simulink model "Hexa_CAD_ANSFT_Sim_V3"  (R2023a)
settings: Solver=ode4  StartTime=0.0  StopTime=30  FixedStep=0.01  RelTol=1e-3
model workspace (MAT data in the model file):
  hover_2m = [0 0 2 0 0 0 0 0 2 0 0 0 ... (36 elements, 6x6)]
  square = [0 0 2.5 0 0 0 0 0 2.5 0 0 0 ... (36 elements, 6x6)]
  tf : Simulink.Parameter (value not decoded)
  tray0 = [0 0 0 0 0 0 0.2 0.15 2 0 0 0 ... (36 elements, 6x6)]
  tray1 = [0 0 0 0 0 0 0 0 2 0 0 0 ... (36 elements, 6x6)]
  tray2 = [0 0 0 0 0 0 2 0 5 0 0 0 ... (36 elements, 6x6)]
  tray3 = [0 0 0 0 0 0 2 0 5 0 0 0 ... (36 elements, 6x6)]
  tray4 = [0 0 0 0 0 0 2 0 5 0.15 0 0 ... (36 elements, 6x6)]
  tray5 = [0 0 0 0 0 0 0 0 5 0.15 0 0 ... (36 elements, 6x6)]
  tray_yaw = [0 0 0 0 0 0 0 0 5 0 0 0 ... (36 elements, 6x6)]
undefined symbols (not defined in the file or in its folder): F, Light, MIL, smiData, X, Y, Z
libraries: sm_lib x168, nesl_utility x33, dspsrcs4 x9, sharedtransform x3, simulink x3, robotcorelib x1, aerolibwind2 x1
(part 6 of 6)

== matlab function Hexa_CAD_ANSFT_Sim_V3/Trajectory/Helicoidal Trajectory ==
  data: time input; pose_d output; pose_d_dot output; pose_d_ddot output
function [pose_d, pose_d_dot, pose_d_ddot]= fcn(time)

% pos_z = time / 12;
f = 0.15;
arg = f * (time - 5);
r = 2;

% hover for 5 s | include inclination in roll
% 5 metros al menos

roll = 0;
% yaw = pi / 2;
yaw = 0;

if (time < 5)
    pos_x = 0;
    pos_y = 0;
    % roll = 0;
    pos_z = 0.4 * time;
    % yaw = 0;
else
    pos_x = -r + r * cos (arg);
    pos_y = r * sin (arg);
    pos_z = 2;
    % roll = 0.15;
    % yaw = (time - 5) * 2 * pi / 180; 
end

% roll = 0;
% yaw = time * 0;

pose_d = [pos_x;
          pos_y;
          pos_z;
          roll;
          0;
          yaw];

% pos_z_dot = 1 / 12;

% hover for 5 s
if (time < 5)
    pos_x_dot = 0;
    pos_y_dot = 0;
    pos_z_dot = 0.4;
    % yaw_dot = 0;
else
    pos_x_dot = - f * r * sin(arg);
    pos_y_dot = f * r * cos(arg);
    pos_z_dot = 0;
    % yaw_dot = 2 * pi / 180;
end

yaw_dot = 0;

pose_d_dot = [pos_x_dot;
              pos_y_dot;
              pos_z_dot;
              0;
              0;
              yaw_dot*0];

pos_z_ddot = 0;
% hover for 5 s
if (time < 5)
    pos_x_ddot = 0;
    pos_y_ddot = 0;
else
    pos_x_ddot = - f * f * r * cos(arg);
    pos_y_ddot = - f * f * r * sin(arg);
end

pose_d_ddot = [pos_x_ddot;
               pos_y_ddot;
               pos_z_ddot;
               0;
               0;
               0];

== matlab function Hexa_CAD_ANSFT_Sim_V3/Controller/ANSFT Constants ==
  data: unused input; xi1 output; xi2 output; lambda1 output; lambda2 output; alpha output; beta output; epsilon output
function [xi1, xi2, lambda1, lambda2, alpha, beta, epsilon] = fcn(~)

%% Constantes de la Superficie deslizante
xi1 = [2.5; 2.5; 1.5; 1; 1; 1];
xi2 = [1.25; 1.25; 2; 0.5; 0.5; 0.5];
lambda1 = [1.5; 1.5; 1.75; 2; 2; 2];
lambda2 = [1.2; 1.2; 1.25; 1.2; 1.2; 1.2];
%% Constantes del control auxiliar
alpha = [1.75; 1.75; 0.625; 2.5; 2.5; 1.25];
beta = [2.5; 2.5; 0.1; 0.05; 0.05; 0.25];
epsilon = [0.4; 0.4; 0.4; 0.2; 0.2; 0.2];

== matlab function Hexa_CAD_ANSFT_Sim_V3/Controller/Constants Functions ==
  data: Phi output; M output; M_inv output; v input
function [Phi, M, M_inv] = fcn(v)

%% system constants
m = 1.8; %5 mass 2.2 kg
Jxx = 0.0393;       % Inercia x.
Jyy = 0.0409;       % Inercia y.
Jzz = 0.0596;       % Inercia z.

%% Phi matrix calculation
uu = v(1);
vv = v(2);
ww = v(3);
pp = v(4);
qq = v(5);
rr = v(6);

Phi = [0, -rr, qq, 0, -ww, vv;
        rr, 0, -pp , ww, 0, -uu;
        -qq, pp, 0,  -vv, uu, 0;
        0, 0, 0, 0, -rr, qq; 
        0, 0, 0, rr, 0, -pp;
        0, 0, 0, -qq, pp, 0];

M = [m, 0, 0, 0, 0, 0;
    0, m, 0, 0, 0, 0;
    0, 0, m, 0, 0, 0;
    0, 0, 0, Jxx, 0, 0;
    0, 0, 0, 0, Jyy, 0;
    0, 0, 0, 0, 0, Jzz];

M_inv = inv(M);

== matlab function Hexa_CAD_ANSFT_Sim_V3/Trajectory/Lemniscate Trajectory ==
  data: time input; pose_d output; pose_d_dot output; pose_d_ddot output
function [pose_d, pose_d_dot, pose_d_ddot]= fcn(time)

%% Positions

arg = time / 4;
rx = 2;
ry = 2;

pos_x = rx * sin(arg);
pos_y = ry * sin(arg) * cos(arg);
pos_z = 0;

yaw = time * 0;

pose_d = [pos_x;
          pos_y;
          pos_z;
          0;
          0;
          yaw];

%% Velocities

pos_x_dot = rx * 0.25 * cos(arg);
pos_y_dot = ry * 0.25 * cos(2 * arg);
pos_z_dot = 0;
yaw_dot = 0;

pose_d_dot = [pos_x_dot;
              pos_y_dot;
              pos_z_dot;
              0;
              0;
              yaw_dot];

%% Accelerations

pos_x_ddot = - rx * 0.25 * 0.25 * sin(arg);
pos_y_ddot = - ry * 0.25 * 0.25 * 2 * sin(arg);
pos_z_ddot = 0;
yaw_ddot = 0;

pose_d_ddot = [pos_x_ddot;
               pos_y_ddot;
               pos_z_ddot;
               0;
               0;
               yaw_ddot];

== matlab function Hexa_CAD_ANSFT_Sim_V3/Controller/Rib function ==
  data: pose input; Rbi output
function Rbi  = fcn(pose)

%% Rib matrix calculation

roll = pose(4);
pitch = pose(5);
yaw = pose(6);

R1 = [cos(yaw)*cos(pitch), -cos(roll)*sin(yaw) + cos(yaw)*sin(roll)*sin(pitch), sin(roll)*sin(yaw) + cos(roll)*cos(yaw)*sin(pitch);
       cos(pitch)*sin(yaw), cos(roll)*cos(yaw) + sin(yaw)*sin(pitch)*sin(roll), -cos(yaw)*sin(roll) + sin(yaw)*sin(pitch)*cos(roll);
       -sin(pitch), cos(pitch)*sin(roll), cos(pitch)*cos(roll)];

R2 = [1, sin(roll)*tan(pitch), cos(roll)*tan(pitch);
      0, cos(roll), -sin(roll);
      0, sin(roll)/cos(pitch), cos(roll)/cos(pitch)];

Rzeros = zeros(3);

Rib = [R1, Rzeros;
       Rzeros, R2];
Rbi = inv(Rib);

== matlab function Hexa_CAD_ANSFT_Sim_V3/6DoF_Dynamics/calculatePWM ==
  data: omega2 input; pwm output
function pwm = fcn(omega2)

pwm = -1.3121e-09 .* omega2 .* omega2 + 0.00208 .* omega2 + 1107.922;

== matlab function Hexa_CAD_ANSFT_Sim_V3/SecondOrderFilter/SOF_gains ==
  data: omega_n output
function omega_n = fcn

omega_n = [30; 30; 50; 70; 50; 50];
